simulink model "PneumaticActOpenLoop"  (R2018b)
settings: Solver=ode15s  StartTime=0.0  StopTime=2  RelTol=1e-3
PreLoadFcn:
  | pneumaticInitialization
  | parametersMultibody
values from neighbouring files (symbols this model uses):
  base_breadth = 1    [parametersMultibody.m]
  base_height = 0.05    [parametersMultibody.m]
  base_length = 3.5    [parametersMultibody.m]
  box_breadth = 0.03    [parametersMultibody.m]
  box_height = 0.005    [parametersMultibody.m]
  box_height_s = 0.002    [parametersMultibody.m]
  box_length = 0.03    [parametersMultibody.m]
  box_yellow_breadth = 0.3    [parametersMultibody.m]
  box_yellow_height = 0.02    [parametersMultibody.m]
  box_yellow_length = 0.2    [parametersMultibody.m]
  frame_stand_breadth = 0.02    [parametersMultibody.m]
  frame_stand_height = 0.4280    (= 0.428)    [parametersMultibody.m]
  frame_stand_length = 0.02    [parametersMultibody.m]
undefined symbols (not defined in the file or in its folder): A_pipe, A_piston, delta_p, L_pipe, L_piston, p_init, sigbuilder_block, T_init, X, Y, Z
libraries: sm_lib x51, fl_lib x33, Contact_Forces_Lib x15, nesl_utility x7, Multibody_Parts_Lib x2, SimscapeFluids_lib x1, sm_backhoe_lib x1, simulink x1
(part 1 of 4)
settings Model: Creator=valakshe  LastModifiedBy=valakshe
settings SolverCC: MaxOrder=2  ZeroCrossAlgorithm=Adaptive
settings DataIOCC: ReturnWorkspaceOutputsName=tpc4ffeed1_4cd0_47cf_96e6_fe3975a5b339
settings OptimizationCC: EfficientMapNaN2IntZero=off
settings DebuggingCC: AlgebraicLoopMsg=none  ArtificialAlgebraicLoopMsg=none  MaxConsecutiveZCsMsg=none  MaskedZcDiagnostic=none  IgnoredZcDiagnostic=none  ModelReferenceExtraNoncontSigs=warning  SimStateInterfaceChecksumMismatchMsg=none  LibraryContextMissingDiagnostic=none
settings HardwareCC: TargetBitPerPointer=64  TargetBitPerSizeT=64  TargetBitPerPtrDiffT=64  TargetLongLongMode=on  TargetIntDivRoundTo=Zero  TargetEndianess=LittleEndian  TargetWordSize=64  TargetHWDeviceType=MATLAB Host  ProdEqTarget=off
settings SFSimCC: SimUseLocalCustomCode=off
settings CodeAppCC: MaxIdLength=128
settings GRTTargetCC: TargetLangStandard=C89/C90 (ANSI)  CombineOutputUpdateFcns=off  GRTInterface=on
settings DiagnosticsConfigSet: SimMechanicsRigidlyBoundBlock=none  SimMechanicsJointTargetOverSpecification=warning
settings ExplorerConfigSet: InternalSimMechanicsExplorerSettings="<ExplorerConfiguration><canonicalview>default</canonicalview><AnimationSetting><BasePlaybackSpeed>1.0</BasePlaybackSpeed><PlaybackSpeedFactor>0.25</PlaybackSpeedFactor></AnimationSetting><TilePanel><TileInfo><Tiles Columns=\"1\" Count=\"1\" Rows=\"1\"><Column Weight=\"1\"/><Row Weight=\"1\"/><Tile Height=\"1\" Width=\"1\" X=\"0\" Y=\"0\"/></Tiles></TileInfo><SceneInfo><SceneViewer><BGColor><R>1</R><G>1</G><B>1</B></BGColor><Camera><DoPerspective>off</DoPerspective><Position><X>2.57635917191157215</X><Y>-0.932254312386120221</Y><Z>0.641449463906099138</Z></Position><Center><X>1.50967147978773308</X><Y>0.134433379737718989</Y><Z>-0.425238228217740211</Z></Center><Up><X>-0.408248290463863073</X><Y>0.408248290463863073</Y><Z>0.816496580927726145</Z></Up><ViewLimDist>1</ViewLimDist><YLim>1.58397085572147422</YLim><XLim>2.39924997263693873</XLim></Camera></SceneViewer></SceneInfo></TilePanel><MechEditorPanel><Cameras/><GfxPanelCameraMap/><VideoCreator><PlaybackSpeedRatio>1.0</PlaybackSpeedRatio><FrameRate>30</FrameRate><VideoFormat>Motion JPEG AVI</VideoFormat><FrameSize>auto</FrameSize></VideoCreator></MechEditorPanel></ExplorerConfiguration>"

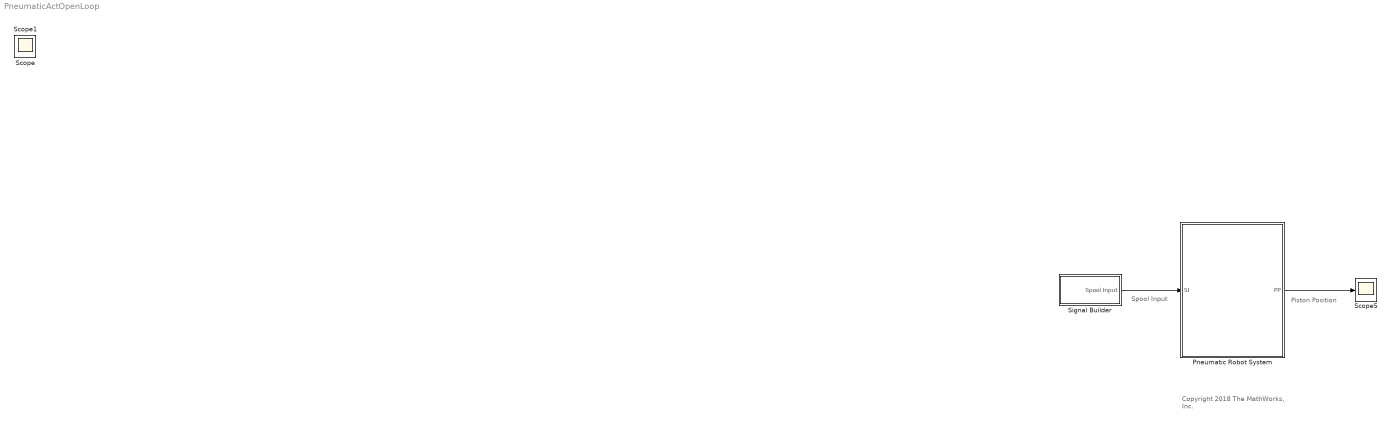
== system PneumaticActOpenLoop ==
  note: Piston Position
  note: Spool Input
  note: Copyright 2018 The MathWorks, Inc.
  Pneumatic Robot System : Subsystem
      mask Display: image("Pneumatic Robot System.png")
  Scope5 : Scope
  Signal Builder : Subsystem  Tag=STV Subsys  LoadFcn=sigbuilder_block('load');  StartFcn=sigbuilder_block('start');  StopFcn=sigbuilder_block('stop');  ClipboardFcn=sigbuilder_block('clipboard');  mask(Sigbuilder block){tuvar=[0:10]}
      mask help: Simulink:masks:SigbuilderBlock_MD
      mask init:
      | if ~strcmp(get_param(bdroot(gcbh),'SimulationStatus'),'stopped') tuvar = sigbuilder_block('maskInit'); end
      settings: CopyFcn=sigbuilder_block('copy');  DeleteFcn=sigbuilder_block('delete');  ModelCloseFcn=sigbuilder_block('modelClose');  PreSaveFcn=sigbuilder_block('preSave');  PauseFcn=sigbuilder_block('pause');  ContinueFcn=sigbuilder_block('continue');  NameChangeFcn=sigbuilder_block('namechange');  OpenFcn=sigbuilder_block('open',[10 -122 550.5 362.5 ]);  CloseFcn=sigbuilder_block('close');
      mask Display: plot(0, 0, 100, 100,[2, 2, 32, 32, 2], [68, 8, 8, 68, 68],[32, 2], [38, 38], [32, 19, 2],[53, 60, 44], [32, 17, 17, 2],[16, 16, 31, 31]);txt = getActiveGroup(gcbh);text(2, 100, txt,'verticalAlignment', 'top');
  Scope : Scope
  Scope1 : Scope
  wires:
  Signal Builder/1(Spool Input) -> Pneumatic Robot System/1(SI)
  Pneumatic Robot System/1(PP) -> Scope5/1

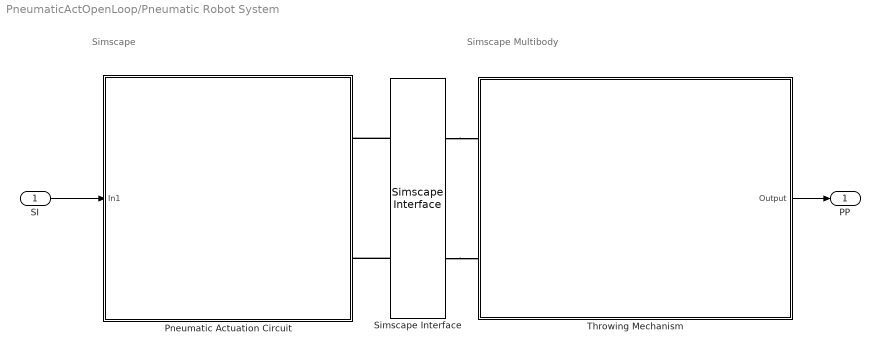
== system PneumaticActOpenLoop/Pneumatic Robot System ==
  note: Simscape
  note: Simscape Multibody
  SI : Inport
  Pneumatic Actuation Circuit : Subsystem
  Simscape Interface : sm_backhoe_lib/Hydraulic Actuator/Simscape Interface  SystemSampleTime=-1
  Throwing Mechanism : Subsystem
      mask Display: image('Simscape_model.jpg')
  PP : Outport
  wires:
  SI/1 -> Pneumatic Actuation Circuit/1(In1)
  Throwing Mechanism/1(Output) -> PP/1
  connections:
  Simscape Interface/RConn1 -- Pneumatic Actuation Circuit/RConn1
  Simscape Interface/RConn2 -- Pneumatic Actuation Circuit/RConn2
  Simscape Interface/LConn1 -- Throwing Mechanism/LConn1
  Simscape Interface/LConn2 -- Throwing Mechanism/LConn2

== system PneumaticActOpenLoop/Signal Builder ==
  Demux : Demux  Tag=STV Demux  Outputs=1
  FromWs : FromWorkspace  Tag=STV FromWs  VariableName=tuvar  SampleTime=0
      SigBuilderData=|
      | common.afterFinalStr = 'Extrapolate'
      | common.sampleTime = 0
      | dataSet.timeRange = [0 4]
      | dataSet.name = 'Group 1'
      | sbobj.Groups.Name = 'Group 1'
      | sbobj.Groups.Signals.Name = 'Spool Input'
      | sbobj.Groups.Signals.XData = [0 0.1 0.1 0.14 0.14 4]
      | sbobj.Groups.Signals.YData = [0 0 0.03 0.03 0 0]
      | sbobj.Groups.TimeRange = [0 4]
  Spool Input : Outport  Tag=STV Outport
  wires:
  FromWs/1 -> Demux/1
  Demux/1 -> Spool Input/1
